simulink model "full_order_as_tf_without_resistances_to_pdf"  (R2015b)
settings: Solver=VariableStepAuto  StartTime=0.0  StopTime=10.0  RelTol=1e-3
undefined symbols (not defined in the file): J_pro, Kt, Kv, R, TS, Vin
settings Model: Creator=Morten  LastModifiedBy=Morten

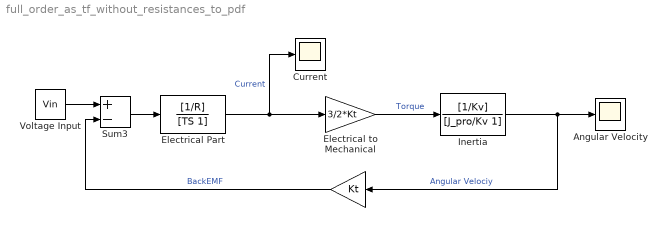
== system full_order_as_tf_without_resistances_to_pdf ==
  "             " : Gain  Gain=Kt
  "Angular Velocity " : Scope
  "Current " : Scope
  "Electrical Part " : TransferFcn  Numerator=[1/R]  Denominator=[TS 1]
  "Electrical to Mechanical " : Gain  Gain=3/2*Kt
  "Inertia " : TransferFcn  Numerator=[1/Kv]  Denominator=[J_pro/Kv 1]
  Sum3 : Sum  Inputs=+-
  "Voltage Input " : Constant  Value=Vin
  wires:
  "             "/1 -> Sum3/2  "BackEMF"
  Sum3/1 -> "Electrical Part "/1
  "Electrical Part "/1 -> "Current "/1, "Electrical to Mechanical "/1  "Current"
  "Voltage Input "/1 -> Sum3/1
  "Electrical to Mechanical "/1 -> "Inertia "/1  "Torque"
  "Inertia "/1 -> "Angular Velocity "/1, "             "/1  "Angular Velociy"
